simulink model "lqr_1dof_nonlinear_force"  (R2017a)
settings: Solver=ode45  StartTime=0.0  StopTime=10  RelTol=1e-3
undefined symbols (not defined in the file): f, g, J, K, L, l, m_p
settings Model: Creator=sansh  LastModifiedBy=rj2318

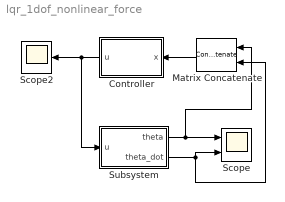
== system lqr_1dof_nonlinear_force ==
  Controller : Subsystem
  Matrix Concatenate : Concatenate  Mode=Multidimensional array  ConcatenateDimension=2
  Scope : Scope  NumInputPorts=2
  Scope2 : Scope
  Subsystem : Subsystem
  wires:
  Controller/1(u) -> Subsystem/1(u), Scope2/1
  Subsystem/1(theta) -> Matrix Concatenate/1, Scope/1
  Subsystem/2(theta_dot) -> Scope/2, Matrix Concatenate/2
  Matrix Concatenate/1 -> Controller/1(x)

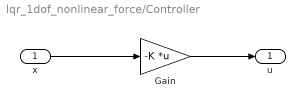
== system lqr_1dof_nonlinear_force/Controller ==
  x : Inport
  Gain : Gain  Gain=-K  Multiplication=Matrix(K*u)
  u : Outport
  wires:
  Gain/1 -> u/1
  x/1 -> Gain/1

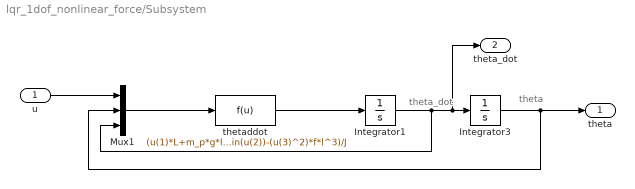
== system lqr_1dof_nonlinear_force/Subsystem ==
  note: theta
  note: theta_dot
  u : Inport
  Integrator1 : Integrator  ContinuousStateAttributes='thetadot'
  Integrator3 : Integrator  InitialCondition=0.1  ContinuousStateAttributes='theta'
  Mux1 : Mux  Inputs=3
  thetaddot : Fcn  Expr=(u(1)*L+m_p*g*l*sin(u(2))-(u(3)^2)*f*l^3)/J
  theta : Outport
  theta_dot : Outport  Port=2
  wires:
  Mux1/1 -> thetaddot/1
  thetaddot/1 -> Integrator1/1
  Integrator1/1 -> Mux1/3, theta_dot/1, Integrator3/1
  Integrator3/1 -> Mux1/2, theta/1
  u/1 -> Mux1/1
